simulink model "LinearHeli"  (R2021a)
settings: Solver=VariableStepAuto  StartTime=0.0  StopTime=10.0  RelTol=1e-3
values from neighbouring files (symbols this model uses):
  Bp = 0.8    [HeliControlGain.m]    (also in HeliControlHinf.m; HeliControlInteger.m; HeliControlIntegerObsv.m; HeliControlLQG.m)
  By = 0.318    [HeliControlGain.m]    (also in HeliControlHinf.m; HeliControlInteger.m; HeliControlIntegerObsv.m; HeliControlLQG.m)
  g = 9.81    [HeliControlGain.m]    (also in HeliControlHinf.m; HeliControlInteger.m; HeliControlIntegerObsv.m; HeliControlLQG.m)
  Jtp = Jeq_p + Mheli*Lcm^2    (= 0.0863915712)    [HeliControlGain.m]    (also in HeliControlHinf.m; HeliControlInteger.m; HeliControlIntegerObsv.m; HeliControlLQG.m)
  Jty = Jeq_y + Mheli*Lcm^2    (= 0.0911915712)    [HeliControlGain.m]    (also in HeliControlHinf.m; HeliControlInteger.m; HeliControlIntegerObsv.m; HeliControlLQG.m)
  Kpp = 0.204    [HeliControlGain.m]    (also in HeliControlHinf.m; HeliControlInteger.m; HeliControlIntegerObsv.m; HeliControlLQG.m)
  Kpy = 0.0068    [HeliControlGain.m]    (also in HeliControlHinf.m; HeliControlInteger.m; HeliControlIntegerObsv.m; HeliControlLQG.m)
  Kyp = 0.0219    [HeliControlGain.m]    (also in HeliControlHinf.m; HeliControlInteger.m; HeliControlIntegerObsv.m; HeliControlLQG.m)
  Kyy = 0.072    [HeliControlGain.m]    (also in HeliControlHinf.m; HeliControlInteger.m; HeliControlIntegerObsv.m; HeliControlLQG.m)
  Lcm = 0.186    [HeliControlGain.m]    (also in HeliControlHinf.m; HeliControlInteger.m; HeliControlIntegerObsv.m; HeliControlLQG.m)
  Mheli = 1.3872    [HeliControlGain.m]    (also in HeliControlHinf.m; HeliControlInteger.m; HeliControlIntegerObsv.m; HeliControlLQG.m)
settings Model: Creator=Ciro  LastModifiedBy=Ciro

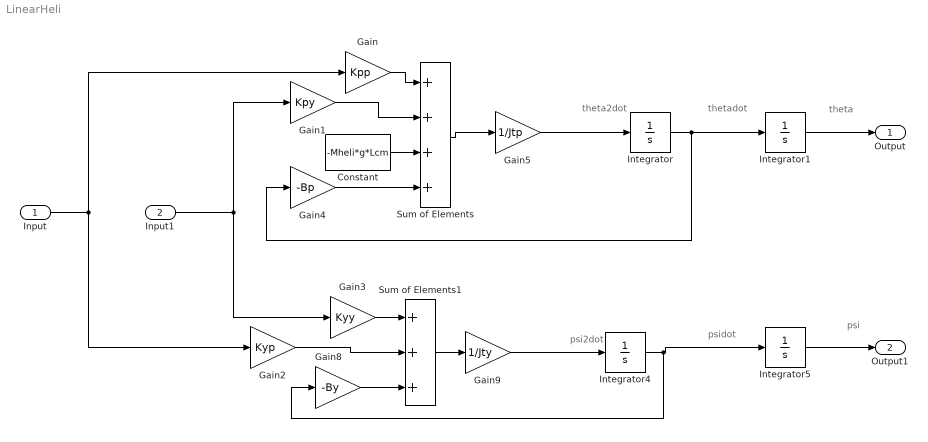
== system LinearHeli ==
  note: psi
  note: theta
  note: thetadot
  note: theta2dot
  note: psidot
  note: psi2dot
  Input : Inport
  Input1 : Inport  Port=2
  Constant : Constant  Value=-Mheli*g*Lcm
  Gain : Gain  Gain=Kpp
  Gain1 : Gain  Gain=Kpy
  Gain2 : Gain  Gain=Kyp
  Gain3 : Gain  Gain=Kyy
  Gain4 : Gain  Gain=-Bp
  Gain5 : Gain  Gain=1/Jtp
  Gain8 : Gain  Gain=-By
  Gain9 : Gain  Gain=1/Jty
  Integrator{,1,4..5} (4 alike) : Integrator
  Sum of Elements : Sum  Inputs=4
  Sum of Elements1 : Sum  Inputs=3
  Output : Outport
  Output1 : Outport  Port=2
  wires:
  Integrator/1 -> Integrator1/1, Gain4/1
  Sum of Elements/1 -> Gain5/1
  Gain/1 -> Sum of Elements/1
  Gain1/1 -> Sum of Elements/2
  Gain4/1 -> Sum of Elements/4
  Constant/1 -> Sum of Elements/3
  Gain9/1 -> Integrator4/1
  Integrator4/1 -> Integrator5/1, Gain8/1
  Gain8/1 -> Sum of Elements1/3
  Gain2/1 -> Sum of Elements1/2
  Gain3/1 -> Sum of Elements1/1
  Input/1 -> Gain2/1, Gain/1
  Input1/1 -> Gain3/1, Gain1/1
  Integrator1/1 -> Output/1
  Integrator5/1 -> Output1/1
  Gain5/1 -> Integrator/1
  Sum of Elements1/1 -> Gain9/1
